simulink model "ctdsm_3OrderFB"  (R2025b)
settings: Solver=VariableStepAuto  StartTime=0.0  StopTime=1  RelTol=1e-6
model workspace (MAT data in the model file):
  DSM_OSR = 64
  DSM_order = 3
  a = [0.0270163801843 0.176750687317 0.573679936448]
  b = [0.0270163801843 0.176750687317 0.573679936448 1]
  c = [1 1 1]
  fs = 128000
  g = 0
libraries: dsphdlfiltering2 x1, dspfdesign x1, dspquant2 x1
settings Model: Creator=The MathWorks, Inc.  LastModifiedBy=sohom
settings RTWCC: LargeConstantGeneration=WriteOnlyDNNConstantsToDataFiles

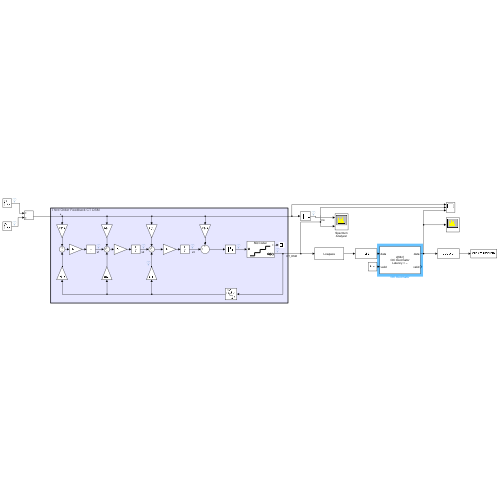
[thumbnail: Simulink's stored preview of the top-level diagram]
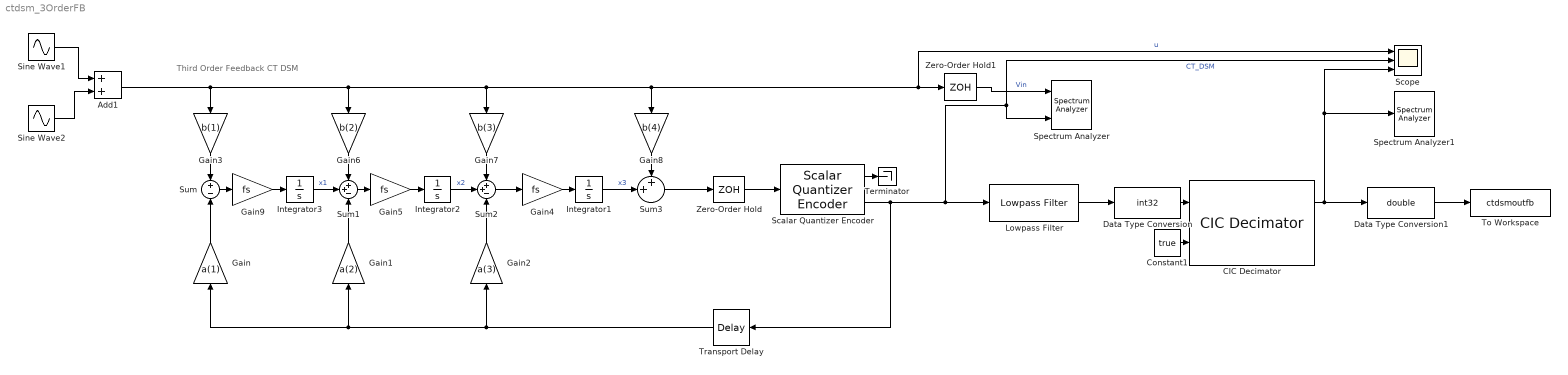
== system ctdsm_3OrderFB ==
  note: Third Order Feedback CT DSM
  Add1 : Sum
  CIC Decimator : dsphdlfiltering2/CIC Decimator  DecimationSource=Property  DecimationFactor=OSR  MaxDecimationFactor=2  DifferentialDelay=1  NumSections=2  GainCorrection=off  SimulateUsing=Code generation  OutputDataType=Full precision  OutputWordLength=16  ResetInputPort=off  HDLGlobalReset=off
  Constant1 : Constant  Value=true
  Data Type Conversion : DataTypeConversion  OutDataTypeStr=int32  SaturateOnIntegerOverflow=off  RndMeth=Floor
  Data Type Conversion1 : DataTypeConversion  OutDataTypeStr=double  SaturateOnIntegerOverflow=off  RndMeth=Floor
  Gain : Gain  Gain=a(1)
  Gain1 : Gain  Gain=a(2)
  Gain2 : Gain  Gain=a(3)
  Gain3 : Gain  Gain=b(1)
  Gain4 : Gain  Gain=fs
  Gain5 : Gain  Gain=fs
  Gain6 : Gain  Gain=b(2)
  Gain7 : Gain  Gain=b(3)
  Gain8 : Gain  Gain=b(4)
  Gain9 : Gain  Gain=fs
  Integrator1 : Integrator
  Integrator2 : Integrator
  Integrator3 : Integrator
  Lowpass Filter : dspfdesign/Lowpass Filter  FilterType=FIR  DesignForMinimumOrder=on  FilterOrder=50  PassbandFrequency=1200  StopbandFrequency=1750  PassbandRipple=0.1  StopbandAttenuation=80  SampleRateMode=Specify on dialog  SampleRate=fs  SimulateUsing=Interpreted execution  roundingMode=Floor  coeffsDataTypeStr=fixdt(1,16)
  Scalar Quantizer Encoder : dspquant2/Scalar Quantizer Encoder  paramSrc=Specify via dialog  partType=Bounded  BBoundary=[-15:2:17]  UBoundary=[2:9]  SearchMethod=Linear  tieBreakRule=Choose the lower index  outQU=on  outQError=off  codebook=[-15:2:15]  outStatus=off  invalidin=Clip  idtype=int8  roundingMode=Floor  overflowMode=off
  Scope : Scope  NumInputPorts=3
      settings: ActiveDisplayYMinimum=-67.890173410404628  ActiveDisplayYMaximum=67.109826589595372
  Sine Wave1 : Sin  Amplitude=0.8*15  Frequency=2*pi*500  SampleTime=0
  Sine Wave2 : Sin  Amplitude=0.1815  Frequency=2*pi*0.99*fs  Phase=pi  SampleTime=0
  Spectrum Analyzer : SpectrumAnalyzer  NumInputPorts=2  WindowPosition=[385.000000,40.000000,766.000000,785.000000,]  Visible=on  ScopeFrameLocation=window  PlotAsTwoSidedSpectrum=off  FrequencyScale=Log  Span=50  CenterFrequency=25  StartFrequency=0  StopFrequency=50  YLimits=[-107.122 65.8696]  ColorLimits=[-20 80]  ShowLegend=on  AllowFFTLengthLessThanSamplesPerUpdate=on  DefaultConfigurationName=spbscopes.SpectrumAnalyzerBlockCfg  IsFrequencyInputMode=0  FrequencyVectorPort=0  FrequencyVectorFromPort=0  FrequencyInputRBWPort=0  FrequencyInputRBWFromPort=0
  Spectrum Analyzer1 : SpectrumAnalyzer  WindowPosition=[368.000000,182.000000,800.000000,500.000000,]  Visible=on  ScopeFrameLocation=window  SampleRate=44.1e3  PlotAsTwoSidedSpectrum=off  FrequencyScale=Log  WindowInvariantSamplesPerUpdate=on  FrequencySpan=Start and stop frequencies  StartFrequency=20  StopFrequency=20e3  YLimits=[32.8932 88.4626]
  Sum : Sum  Inputs=+|-
  Sum1 : Sum  Inputs=++-
  Sum2 : Sum  Inputs=++-
  Sum3 : Sum  Inputs=++|
  Terminator : Terminator
  To Workspace : ToWorkspace  VariableName=ctdsmoutfb  SampleTime=-1
      settings: MaxDataPoints=fs
  Transport Delay : TransportDelay  DelayTime=.05/fs
  Zero-Order Hold : ZeroOrderHold  SampleTime=1/fs
  Zero-Order Hold1 : ZeroOrderHold  SampleTime=1/fs
  wires:
  Scalar Quantizer Encoder/1 -> Terminator/1
  Zero-Order Hold/1 -> Scalar Quantizer Encoder/1
  Sum3/1 -> Zero-Order Hold/1
  Scalar Quantizer Encoder/2 -> Lowpass Filter/1, Scope/2, Spectrum Analyzer/2, Transport Delay/1  "CT_DSM"
  Sum/1 -> Gain9/1
  Transport Delay/1 -> Gain2/1, Gain1/1, Gain/1
  Gain4/1 -> Integrator1/1
  Gain5/1 -> Integrator2/1
  Sum1/1 -> Gain5/1
  Gain/1 -> Sum/2
  Gain3/1 -> Sum/1
  Gain1/1 -> Sum1/3
  Integrator3/1 -> Sum1/2  "x1"
  Integrator2/1 -> Sum2/2  "x2"
  Sum2/1 -> Gain4/1
  Gain2/1 -> Sum2/3
  Gain6/1 -> Sum1/1
  Gain7/1 -> Sum2/1
  Integrator1/1 -> Sum3/2  "x3"
  Gain8/1 -> Sum3/1
  Gain9/1 -> Integrator3/1
  Sine Wave1/1 -> Add1/1
  Sine Wave2/1 -> Add1/2
  Zero-Order Hold1/1 -> Spectrum Analyzer/1  "Vin"
  Add1/1 -> Gain3/1, Gain6/1, Gain8/1, Scope/1, Zero-Order Hold1/1, Gain7/1  "u"
  Constant1/1 -> CIC Decimator/2
  Data Type Conversion/1 -> CIC Decimator/1
  CIC Decimator/1 -> Scope/3, Spectrum Analyzer1/1, Data Type Conversion1/1
  Lowpass Filter/1 -> Data Type Conversion/1
  Data Type Conversion1/1 -> To Workspace/1
